simulink model "Es0_att_dyn_sim"  (R2025b)
settings: Solver=VariableStepAuto  StartTime=0.0  StopTime=60  RelTol=1e-3
values from neighbouring files (symbols this model uses):
  I_B_kgm2 = diag([10 15 20])    [main_att_dyn.m]
  M_ext_B_Nm = 0    [main_att_dyn.m]
  omega_BN_B_Init_radps = [0.0; 0.1; 0.2]    [main_att_dyn.m]
  q_NB_Init = 0.5*ones(4,1)    [main_att_dyn.m]
libraries: matrix_library x1
settings Model: Creator=aayan  LastModifiedBy=aayan

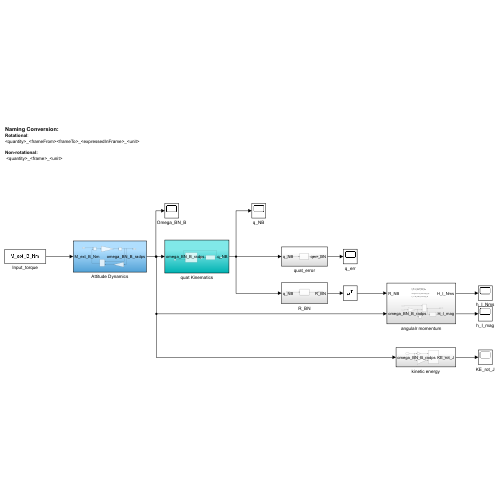
[thumbnail: Simulink's stored preview of the top-level diagram]
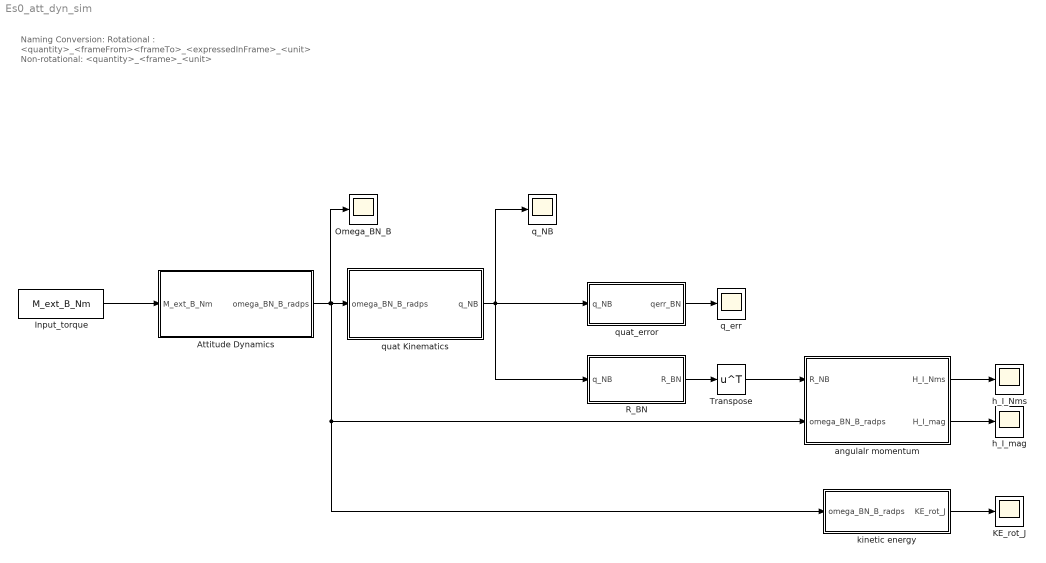
== system Es0_att_dyn_sim ==
  note: Naming Conversion:
      | Rotational :
      | <quantity>_<frameFrom><frameTo>_<expressedInFrame>_<unit>
      |
      | Non-rotational:
      | <quantity>_<frame>_<unit>
  Attitude Dynamics : Subsystem
  Input_torque : Constant  Value=M_ext_B_Nm
  KE_rot_J : Scope
      settings: ActiveDisplayYMinimum=-1  ActiveDisplayYMaximum=1  DataLoggingVariableName=ScopeData5
  Omega_BN_B : Scope
      settings: ActiveDisplayYMinimum=-0.13851036093265784  ActiveDisplayYMaximum=0.24778058919440313  DataLoggingVariableName=ScopeData2
  R_BN : Subsystem
  Transpose : Math  Operator=transpose
  angulalr momentum : Subsystem
  h_I_Nms : Scope
      settings: ActiveDisplayYMinimum=-0.50000000179412241  ActiveDisplayYMaximum=4.5000000161471014  DataLoggingVariableName=ScopeData3
  h_I_mag : Scope
      settings: ActiveDisplayYMinimum=4.2720018301580422  ActiveDisplayYMaximum=4.2720018819533614  DataLoggingVariableName=ScopeData4
  kinetic energy : Subsystem
  q_NB : Scope
      settings: ActiveDisplayYMinimum=-0.99892748538637788  ActiveDisplayYMaximum=1.0695401343709785
  q_err : Scope
      settings: ActiveDisplayYMinimum=-4.0245584642661925E-16  ActiveDisplayYMaximum=2.9143354396410359E-16
  quat Kinematics : Subsystem
  quat_error : Subsystem
  wires:
  Input_torque/1 -> Attitude Dynamics/1(M_ext_B_Nm)
  Attitude Dynamics/1(omega_BN_B_radps) -> kinetic energy/1(omega_BN_B_radps), angulalr momentum/2(omega_BN_B_radps), quat Kinematics/1(omega_BN_B_radps), Omega_BN_B/1
  quat Kinematics/1(q_NB) -> R_BN/1(q_NB), quat_error/1(q_NB), q_NB/1
  quat_error/1(qerr_BN) -> q_err/1
  R_BN/1(R_BN) -> Transpose/1
  Transpose/1 -> angulalr momentum/1(R_NB)
  angulalr momentum/2(H_I_mag) -> h_I_mag/1
  angulalr momentum/1(H_I_Nms) -> h_I_Nms/1
  kinetic energy/1(KE_rot_J) -> KE_rot_J/1

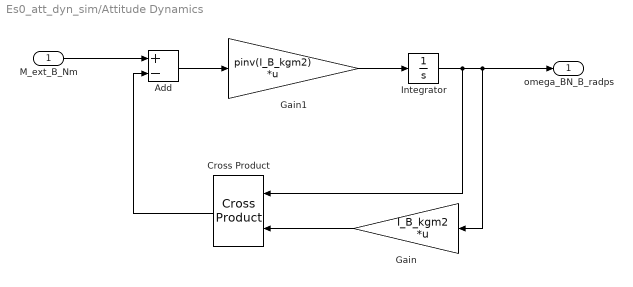
== system Es0_att_dyn_sim/Attitude Dynamics ==
  M_ext_B_Nm : Inport
  Add : Sum  Inputs=+-
  Cross Product : matrix_library/Cross Product
  Gain : Gain  Gain=I_B_kgm2  Multiplication=Matrix(K*u)
  Gain1 : Gain  Gain=pinv(I_B_kgm2)  Multiplication=Matrix(K*u)
  Integrator : Integrator  InitialCondition=omega_BN_B_Init_radps
  omega_BN_B_radps : Outport
  wires:
  M_ext_B_Nm/1 -> Add/1
  Cross Product/1 -> Add/2
  Integrator/1 -> Cross Product/1, Gain/1, omega_BN_B_radps/1
  Gain/1 -> Cross Product/2
  Add/1 -> Gain1/1
  Gain1/1 -> Integrator/1

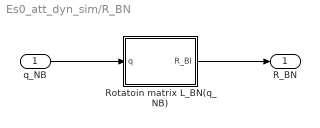
== system Es0_att_dyn_sim/R_BN ==
  q_NB : Inport
  Rotatoin matrix L_BN(q_NB) : MATLAB Function  TreatAsAtomicUnit=on
  R_BN : Outport
  wires:
  q_NB/1 -> Rotatoin matrix L_BN(q_NB)/1(q)
  Rotatoin matrix L_BN(q_NB)/1(R_BI) -> R_BN/1

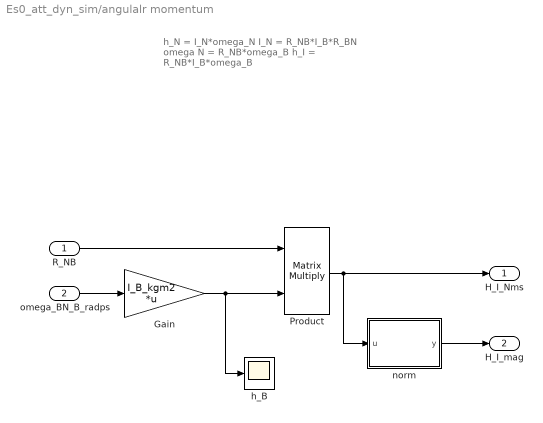
== system Es0_att_dyn_sim/angulalr momentum ==
  note: h_N = I_N*omega_N
      | I_N = R_NB*I_B*R_BN
      |
      | omega N = R_NB*omega_B
      |
      | h_I = R_NB*I_B*omega_B
  R_NB : Inport
  omega_BN_B_radps : Inport  Port=2
  Gain : Gain  Gain=I_B_kgm2  Multiplication=Matrix(K*u)
  Product : Product  Multiplication=Matrix(*)
  h_B : Scope
      settings: ActiveDisplayYMinimum=-2.2083750978534282  ActiveDisplayYMaximum=4.8931859926880925  DataLoggingVariableName=ScopeData6
  norm : MATLAB Function  TreatAsAtomicUnit=on
  H_I_Nms : Outport
  H_I_mag : Outport  Port=2
  wires:
  norm/1(y) -> H_I_mag/1
  Product/1 -> norm/1(u), H_I_Nms/1
  omega_BN_B_radps/1 -> Gain/1
  Gain/1 -> h_B/1, Product/2
  R_NB/1 -> Product/1

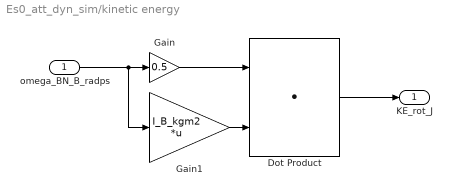
== system Es0_att_dyn_sim/kinetic energy ==
  omega_BN_B_radps : Inport
  Dot Product : DotProduct  OutDataTypeStr=Inherit: Inherit via internal rule
  Gain : Gain  Gain=0.5
  Gain1 : Gain  Gain=I_B_kgm2  Multiplication=Matrix(K*u)
  KE_rot_J : Outport
  wires:
  Gain/1 -> Dot Product/1
  omega_BN_B_radps/1 -> Gain1/1, Gain/1
  Gain1/1 -> Dot Product/2
  Dot Product/1 -> KE_rot_J/1

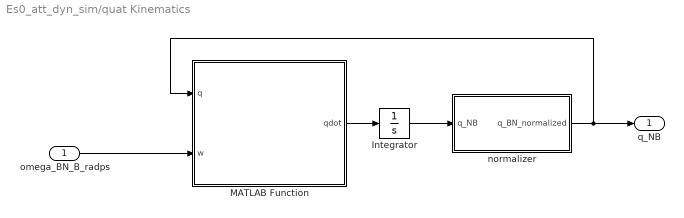
== system Es0_att_dyn_sim/quat Kinematics ==
  omega_BN_B_radps : Inport
  Integrator : Integrator  InitialCondition=q_NB_Init
  MATLAB Function : MATLAB Function  TreatAsAtomicUnit=on
  normalizer : MATLAB Function  TreatAsAtomicUnit=on
  q_NB : Outport
  wires:
  omega_BN_B_radps/1 -> MATLAB Function/2(w)
  MATLAB Function/1(qdot) -> Integrator/1
  Integrator/1 -> normalizer/1(q_NB)
  normalizer/1(q_BN_normalized) -> q_NB/1, MATLAB Function/1(q)

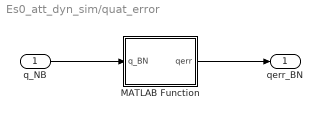
== system Es0_att_dyn_sim/quat_error ==
  q_NB : Inport
  MATLAB Function : MATLAB Function  TreatAsAtomicUnit=on
  qerr_BN : Outport
  wires:
  q_NB/1 -> MATLAB Function/1(q_BN)
  MATLAB Function/1(qerr) -> qerr_BN/1

== matlab function Es0_att_dyn_sim/quat Kinematics/MATLAB Function ==
  data: q input; qdot output; w input
function qdot = fcn(q,w)


W = [ 0    -w(1)   -w(2)   -w(3);
     w(1)    0      w(3)   -w(2);
     w(2)  -w(3)     0      w(1);
     w(3)   w(2)   -w(1)      0];
qdot = 0.5*W*q;

== matlab function Es0_att_dyn_sim/quat_error/MATLAB Function ==
  data: q_BN input; qerr output
function qerr = fcn(q_BN)
qv = q_BN(2:4);
qerr = q_BN(1)^2+qv'*qv-1;

== matlab function Es0_att_dyn_sim/R_BN/Rotatoin matrix L_BN(q_NB) ==
  data: q input; R_BI output
 function R_BI = fcn(q)
q0 = q(1);
qv = q(2:4);

Q_tilde = [  0   -q(4)   q(3);
            q(4)    0   -q(2);
           -q(3)  q(2)    0  ];
R_BI = (q0^2-qv'*qv)*eye(3) + 2*qv*qv'-2*q0*Q_tilde;

== matlab function Es0_att_dyn_sim/angulalr momentum/norm ==
  data: u input; y output
function y = norm(u)

y = sqrt(u(1)^2 + u(2)^2 + u(3)^2);

== matlab function Es0_att_dyn_sim/quat Kinematics/normalizer ==
  data: q_NB input; q_BN_normalized output
function q_BN_normalized = fcn(q_NB)

q_norm = sqrt(q_NB(1)^2+q_NB(2)^2+q_NB(3)^2+q_NB(4)^2);

q_BN_normalized = q_NB/q_norm;
